simulink model "splittedMCU"  (R2021b)
settings: Solver=ode23tb  StartTime=0.0  StopTime=0.06  MaxStep=2.5e-7  RelTol=1e-3  EnableMultiTasking=on
libraries: spsIGBTDiodeLib x6, spsVoltageMeasurementLib x4, spsCurrentMeasurementLib x3, spsMeanLib x3, spsSeriesRLCBranchLib x3, simulink x2, spsControlledVoltageSourceLib x1, spsTHDLib x1, spspowerguiLib x1
settings Model: Creator=Алексей  LastModifiedBy=Len_comp
settings SolverCC: ZeroCrossControl=DisableAll  ZeroCrossAlgorithm=Adaptive  AlgebraicLoopSolver=TrustRegion
settings DataIOCC: SaveFormat=Array  SaveOutput=off  DSMLogging=off  SaveTime=off  ReturnWorkspaceOutputs=off
settings OptimizationCC: LifeSpan=inf
settings DebuggingCC: UnderspecifiedInitializationDetection=Classic  MergeDetectMultiDrivingBlocksExec=none  SolverPrmCheckMsg=warning  AllowSymbolicDim=off  SFUnexpectedBacktrackingDiag=warning  SFNoUnconditionalDefaultTransitionDiag=warning  SFExecutionAtInitializationDiag=none  SFMachineParentedDataDiag=warning  ArithmeticOperatorsInVariantConditions=warning
settings HardwareCC: ProdBitPerPointer=32  ProdBitPerSizeT=32  ProdBitPerPtrDiffT=32  ProdLargestAtomicFloat=None  ProdIntDivRoundTo=Undefined  ProdEndianess=Unspecified  ProdWordSize=32  ProdHWDeviceType=32-bit Generic
settings ModelReferenceCC: PropagateSignalLabelsOutOfModel=off
settings SFSimCC: SimUseLocalCustomCode=off  CustomCodeUndefinedFunction=UseInterfaceOnly
settings RTWCC: RTWUseLocalCustomCode=off
settings CodeAppCC: StateflowObjectComments=on
settings GRTTargetCC: TargetLangStandard=C89/C90 (ANSI)
settings ConfigComp: CovMetricSettings=dw  CovSaveCumulativeToWorkspaceVar=on  CovSaveSingleToWorkspaceVar=on  CovExternalEMLEnable=off  CovSFcnEnable=off
settings SimscapeCC: SimscapeNormalizeSystem=off

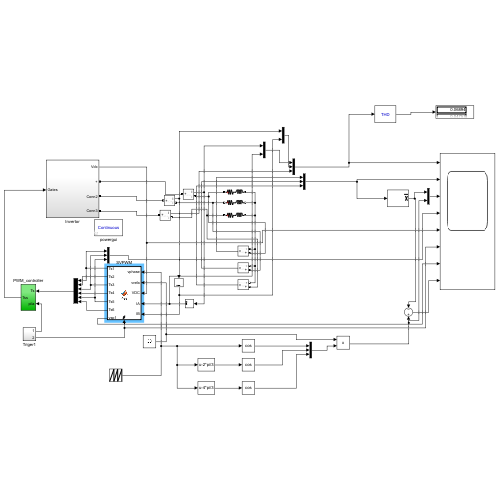
[thumbnail: Simulink's stored preview of the top-level diagram]
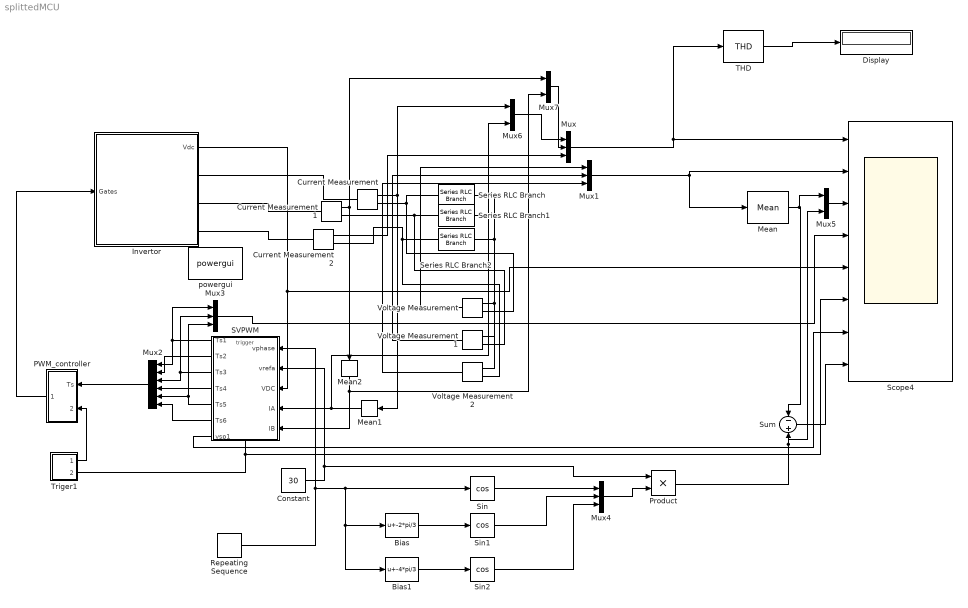
== system splittedMCU ==
  Bias : Bias  Bias=-2*pi/3
  Bias1 : Bias  Bias=-4*pi/3
  Constant : Constant  Value=30
  Current Measurement : spsCurrentMeasurementLib/Current Measurement  PhasorSimulation=off  OutputType=Complex  PSBequivalent=0
  Current Measurement1 : spsCurrentMeasurementLib/Current Measurement  PhasorSimulation=off  OutputType=Complex  PSBequivalent=0
  Current Measurement2 : spsCurrentMeasurementLib/Current Measurement  PhasorSimulation=off  OutputType=Complex  PSBequivalent=0
  Display : Display
  Invertor : Subsystem
  Mean : spsMeanLib/Mean  Freq=50e3  Vinit=0  Ts=0
  Mean1 : spsMeanLib/Mean  Freq=50e3  Vinit=0  Ts=0
  Mean2 : spsMeanLib/Mean  Freq=50e3  Vinit=0  Ts=0
  Mux{,1,3..4} (4 alike) : Mux  Inputs=3
  Mux2 : Mux  Inputs=6
  Mux5 : Mux  Inputs=2
  Mux6 : Mux  Inputs=2
  Mux7 : Mux  Inputs=2
  PWM_controller : Subsystem
  Product : Product
  Repeating Sequence : simulink/Sources/Repeating Sequence  rep_seq_t=[0 0.02]  rep_seq_y=[0 2*pi]
  SVPWM : MATLAB Function  TreatAsAtomicUnit=on
  Scope4 : Scope  NumInputPorts=8
  Series RLC Branch : spsSeriesRLCBranchLib/Series RLC Branch  LConnTagsString=__new0  RConnTagsString=__new0  BranchType=RL  Resistance=1  Inductance=35e-6  SetiL0=off  InitialCurrent=236  Capacitance=1e-6  Setx0=off  InitialVoltage=0  Measurements=None
  Series RLC Branch1 : spsSeriesRLCBranchLib/Series RLC Branch  LConnTagsString=__new0  RConnTagsString=__new0  BranchType=RL  Resistance=1  Inductance=35e-6  SetiL0=off  InitialCurrent=236  Capacitance=1e-6  Setx0=off  InitialVoltage=0  Measurements=None
  Series RLC Branch2 : spsSeriesRLCBranchLib/Series RLC Branch  LConnTagsString=__new0  RConnTagsString=__new0  BranchType=RL  Resistance=1  Inductance=35e-6  SetiL0=off  InitialCurrent=-236  Capacitance=1e-6  Setx0=off  InitialVoltage=0  Measurements=None
  Sin : Trigonometry  Operator=cos
  Sin1 : Trigonometry  Operator=cos
  Sin2 : Trigonometry  Operator=cos
  Sum : Sum  Inputs=-+
  THD : spsTHDLib/THD  Freq=50  Ts=0
      settings: SourceProductBaseCode=PS
  Triger1 : Subsystem
  Voltage Measurement : spsVoltageMeasurementLib/Voltage Measurement  PhasorSimulation=off  OutputType=Complex  PSBequivalent=0
  Voltage Measurement1 : spsVoltageMeasurementLib/Voltage Measurement  PhasorSimulation=off  OutputType=Complex  PSBequivalent=0
  Voltage Measurement2 : spsVoltageMeasurementLib/Voltage Measurement  PhasorSimulation=off  OutputType=Complex  PSBequivalent=0
  powergui : spspowerguiLib/powergui  Priority=1  SimulationMode=Continuous  SampleTime=50e-6  frequency=60  Iterations=50  frequencyindice=0  Pbase=100e6  ErrMax=1e-4  UnitsV=kV  UnitsW=MW  buscounter=0  FunctionMessages=off  echomessages=off  EnableUseOfTLC=off  CurrentSourceSwitches=on  DisableSnubberDevices=off  DisableRonSwitches=off  DisableVfSwitches=off  DisplayEquations=off  AutomaticDiscreteSolvers=off  SolverType=Tustin  Interpol=off  ExternalGateDelay=off  methode=off  Ts=0  x0status=blocks  SPID=off  SwTol=0  HookPort=off  NonlinearTolerance=1e-4  nMaxIteration=100  ContinueOnMaxIteration=off  RestoreLinks=warning  ResistiveCurrentMeasurement=off  Frange=[0:2:500]  Ylog=off  Xlog=on  ShowGrid=off  save=off  variable=ZData  structure=SD2  ZoomFFT=on  StartTime=0.7  cycles=10  DisplayStyle=4  fundamental=382  FreqAxis=off  MaxFrequency=50000  frequencyindicesteady=1  RmsSteady=1  display=off
  wires:
  Mux2/1 -> PWM_controller/1(Ts)
  Triger1/1(1) -> PWM_controller/2(pila)
  PWM_controller/1(Tss) -> Invertor/1(Gates)
  Invertor/1(Vdc) -> Scope4/5, SVPWM/3(VDC)
  SVPWM/1(Ts1) -> Mux2/1, Mux3/1
  SVPWM/2(Ts2) -> Mux2/2
  SVPWM/3(Ts3) -> Mux2/3, Mux3/2
  SVPWM/4(Ts4) -> Mux2/4
  SVPWM/5(Ts5) -> Mux3/3, Mux2/5
  SVPWM/6(Ts6) -> Mux2/6
  Triger1/2(2) -> Scope4/6, SVPWM/Trigger
  Current Measurement/1 -> Mux6/1, Mean1/1
  Current Measurement1/1 -> Mux7/1, Mean2/1
  Constant/1 -> Product/1, SVPWM/2(vrefa)
  Repeating Sequence/1 -> Bias1/1, Bias/1, Sin/1, SVPWM/1(vphase)
  Current Measurement2/1 -> Mux/3
  Mux/1 -> THD/1, Scope4/1
  Voltage Measurement/1 -> Mux1/1
  Voltage Measurement1/1 -> Mux1/2
  Voltage Measurement2/1 -> Mux1/3
  Mean/1 -> Mux5/1, Sum/1
  Mux1/1 -> Mean/1, Scope4/2
  Mux3/1 -> Scope4/4
  SVPWM/7(vsp1) -> Scope4/7
  THD/1 -> Display/1
  Bias/1 -> Sin1/1
  Bias1/1 -> Sin2/1
  Sin/1 -> Mux4/1
  Sin1/1 -> Mux4/2
  Sin2/1 -> Mux4/3
  Mux4/1 -> Product/2
  Product/1 -> Mux5/2, Sum/2
  Sum/1 -> Scope4/8
  Mean1/1 -> Mux6/2, SVPWM/4(IA)
  Mean2/1 -> SVPWM/5(IB), Mux7/2
  Mux5/1 -> Scope4/3
  Mux6/1 -> Mux/1
  Mux7/1 -> Mux/2
  connections:
  Current Measurement/LConn1 -- Invertor/RConn1
  Invertor/RConn3 -- Current Measurement2/LConn1
  Invertor/RConn2 -- Current Measurement1/LConn1
  Voltage Measurement/LConn2 -- Voltage Measurement2/LConn2 -- Voltage Measurement1/LConn2 -- Series RLC Branch/RConn1 -- Series RLC Branch1/RConn1 -- Series RLC Branch2/RConn1
  Current Measurement/RConn1 -- Series RLC Branch/LConn1 -- Voltage Measurement/LConn1
  Current Measurement1/RConn1 -- Series RLC Branch1/LConn1 -- Voltage Measurement1/LConn1
  Current Measurement2/RConn1 -- Series RLC Branch2/LConn1 -- Voltage Measurement2/LConn1

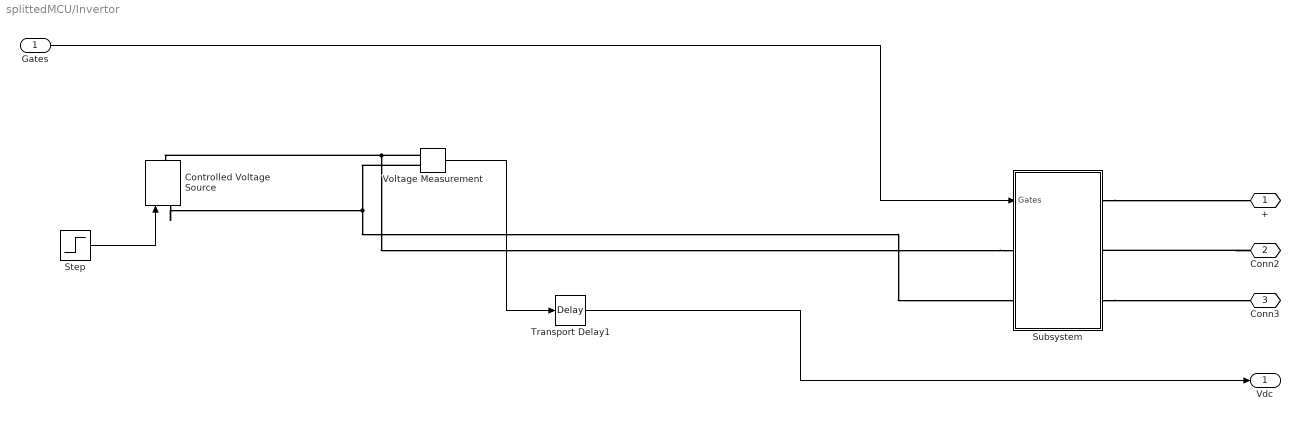
== system splittedMCU/Invertor ==
  Gates : Inport
  Controlled Voltage Source : spsControlledVoltageSourceLib/Controlled Voltage Source  Initialize=on  Source_Type=AC  Amplitude=0  Phase=0  Frequency=0  Measurements=None
  Step : Step  Time=6  Before=100  After=300  SampleTime=0
  Subsystem : Subsystem
  Transport Delay1 : TransportDelay  DelayTime=26e-6
  Voltage Measurement : spsVoltageMeasurementLib/Voltage Measurement  PhasorSimulation=off  OutputType=Complex  PSBequivalent=0
  + : PMIOPort  Side=Right
  Conn2 : PMIOPort  Port=2  Side=Right
  Conn3 : PMIOPort  Port=3  Side=Right
  Vdc : Outport  VectorParamsAs1DForOutWhenUnconnected=off
  wires:
  Voltage Measurement/1 -> Transport Delay1/1
  Transport Delay1/1 -> Vdc/1
  Step/1 -> Controlled Voltage Source/1
  Gates/1 -> Subsystem/1(Gates)
  connections:
  Subsystem/LConn1 -- Controlled Voltage Source/RConn1 -- Voltage Measurement/LConn1
  Subsystem/RConn1 -- +/RConn1
  Conn2/RConn1 -- Subsystem/RConn2
  Subsystem/RConn3 -- Conn3/RConn1
  Voltage Measurement/LConn2 -- Controlled Voltage Source/LConn1 -- Subsystem/LConn2

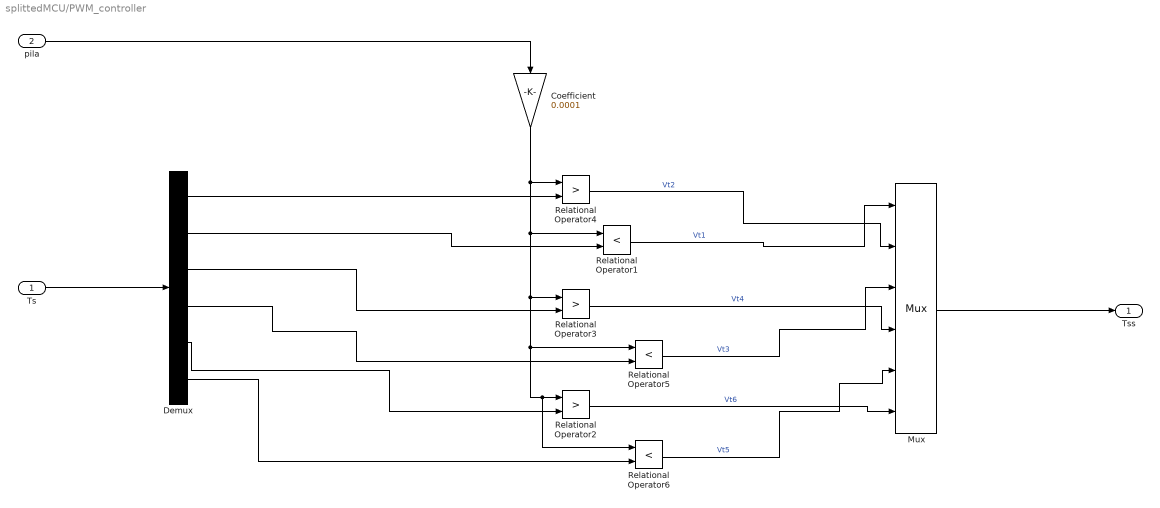
== system splittedMCU/PWM_controller ==
  Ts : Inport
  pila : Inport  Port=2
  Coefficient : Gain  Gain=0.0001
  Demux : Demux  Outputs=6
  Mux : Mux  Inputs=6
  Relational Operator1 : RelationalOperator  Operator=<  OutDataTypeStr=boolean  RndMeth=Nearest
  Relational Operator2 : RelationalOperator  Operator=>  OutDataTypeStr=boolean  RndMeth=Nearest
  Relational Operator3 : RelationalOperator  Operator=>  OutDataTypeStr=boolean  RndMeth=Nearest
  Relational Operator4 : RelationalOperator  Operator=>  OutDataTypeStr=boolean  RndMeth=Nearest
  Relational Operator5 : RelationalOperator  Operator=<  OutDataTypeStr=boolean  RndMeth=Nearest
  Relational Operator6 : RelationalOperator  Operator=<  OutDataTypeStr=boolean  RndMeth=Nearest
  Tss : Outport  VectorParamsAs1DForOutWhenUnconnected=off
  wires:
  Relational Operator4/1 -> Mux/2  "Vt2"
  Demux/3 -> Relational Operator3/2
  Demux/5 -> Relational Operator2/2
  Relational Operator3/1 -> Mux/4  "Vt4"
  Relational Operator2/1 -> Mux/6  "Vt6"
  Ts/1 -> Demux/1
  Coefficient/1 -> Relational Operator1/1, Relational Operator3/1, Relational Operator5/1, Relational Operator6/1, Relational Operator2/1, Relational Operator4/1
  Relational Operator1/1 -> Mux/1  "Vt1"
  Relational Operator5/1 -> Mux/3  "Vt3"
  Relational Operator6/1 -> Mux/5  "Vt5"
  Demux/2 -> Relational Operator1/2
  Demux/4 -> Relational Operator5/2
  Demux/6 -> Relational Operator6/2
  Demux/1 -> Relational Operator4/2
  pila/1 -> Coefficient/1
  Mux/1 -> Tss/1

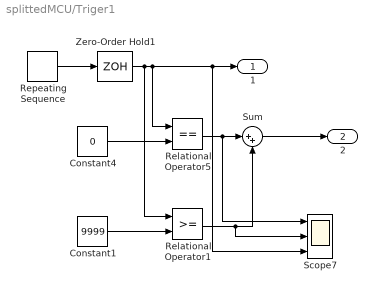
== system splittedMCU/Triger1 ==
  Constant1 : Constant  Value=9999
  Constant4 : Constant  Value=0
  Relational Operator1 : RelationalOperator  OutDataTypeStr=boolean  RndMeth=Nearest
  Relational Operator5 : RelationalOperator  Operator===  OutDataTypeStr=boolean  RndMeth=Nearest
  Repeating Sequence : simulink/Sources/Repeating Sequence  rep_seq_t=[0 10e-6 20e-6]  rep_seq_y=[0 10000 0]
  Scope7 : Scope  NumInputPorts=3
  Sum : Sum  Inputs=|++
  Zero-Order Hold1 : ZeroOrderHold  SampleTime=2.5e-8
  1 : Outport  VectorParamsAs1DForOutWhenUnconnected=off
  2 : Outport  Port=2  VectorParamsAs1DForOutWhenUnconnected=off
  wires:
  Zero-Order Hold1/1 -> Relational Operator1/1, Relational Operator5/1, Scope7/3, 1/1
  Repeating Sequence/1 -> Zero-Order Hold1/1
  Constant4/1 -> Relational Operator5/2
  Sum/1 -> 2/1
  Constant1/1 -> Relational Operator1/2
  Relational Operator5/1 -> Scope7/1, Sum/1
  Relational Operator1/1 -> Scope7/2, Sum/2

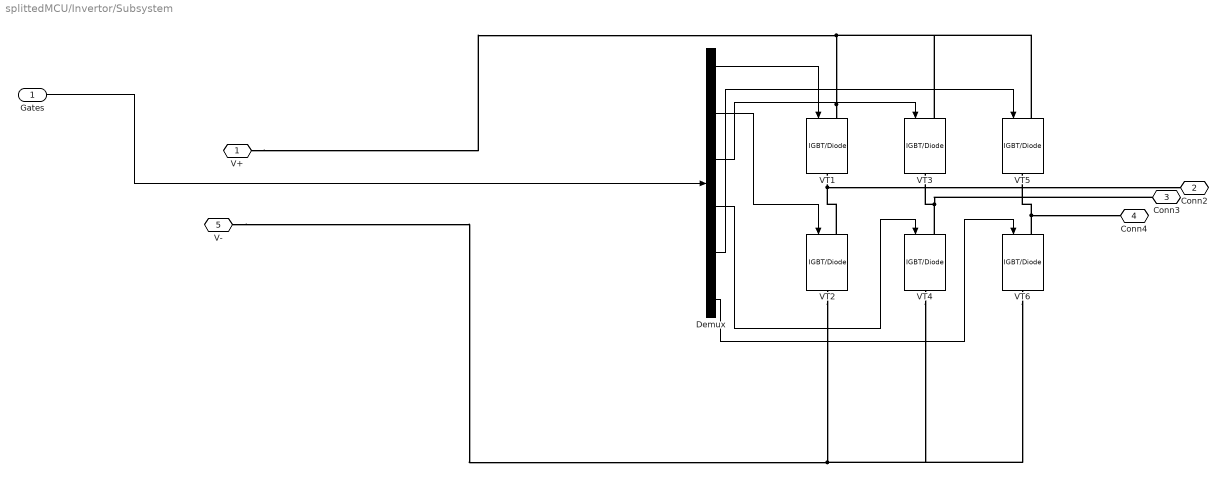
== system splittedMCU/Invertor/Subsystem ==
  Gates : Inport
  Demux : Demux  Outputs=6
  VT{1..6} (6 alike) : spsIGBTDiodeLib/IGBT//Diode  Ron=1e-3  Rs=1e5  Cs=inf  Measurements=off
  V+ : PMIOPort  Side=Left
  Conn2 : PMIOPort  Port=2  Side=Right
  Conn3 : PMIOPort  Port=3  Side=Right
  Conn4 : PMIOPort  Port=4  Side=Right
  V- : PMIOPort  Port=5  Side=Left
  wires:
  Demux/4 -> VT4/1
  Demux/2 -> VT2/1
  Demux/5 -> VT5/1
  Demux/3 -> VT3/1
  Demux/6 -> VT6/1
  Demux/1 -> VT1/1
  Gates/1 -> Demux/1
  connections:
  VT6/LConn1 -- Conn4/RConn1 -- VT5/RConn1
  V-/RConn1 -- VT2/RConn1 -- VT4/RConn1 -- VT6/RConn1
  VT4/LConn1 -- Conn3/RConn1 -- VT3/RConn1
  VT1/LConn1 -- V+/RConn1 -- VT5/LConn1 -- VT3/LConn1
  VT2/LConn1 -- Conn2/RConn1 -- VT1/RConn1

== matlab function splittedMCU/SVPWM ==
  data: vphase input; vrefa input; VDC input; IA input; IB input; Ts1 output; Ts2 output; Ts3 output; Ts4 output; Ts5 output; Ts6 output; vsp1 output
  events: trigger input RISING_EDGE_EVENT
function [Ts1,Ts2,Ts3,Ts4,Ts5,Ts6,vsp1] = fcn(vphase,vrefa,VDC,IA,IB)
%время 1/2 ШИМ периода
dt=10e-6;


%алгоритм формирования векторной ШИМ  мертвым веменем dead [мкс]
dead=1.5;

compensate = 1;


vsp1 = vphase;

dead=dead/(dt*1e6);
a=vphase;
v2=vrefa*1.5;
if a>=0 && a<pi/3 
    n=1;
elseif  a>=pi/3 && a<2*pi/3 
    n=2;
elseif  a>=2*pi/3 && a<pi 
    n=3;
elseif  a>=pi && a<4*pi/3 
    n=4;
elseif  a>=4*pi/3 && a<5*pi/3 
    n=5;
else n=6;

end

a_cor=a-(n-1)*pi/3;

T1 = (v2/VDC)*sin(pi/3-a_cor)/sin(pi/3);
T2 = (v2/VDC)*sin(a_cor)/sin(pi/3);
T0=1-T1-T2;
Ta1=0; Ta3=0; Ta5=0; 
switch n
    case 1
        
        Ta1=T1+T2+T0/2;
        
        Ta3=T2+T0/2;
       
        Ta5=T0/2;
       
    case 2
        
        Ta1=T1+T0/2;
        
        Ta3=T1+T2+T0/2;
    
        Ta5=T0/2;       
        
    case 3
        
        Ta1=T0/2;
       
        Ta3=T1+T2+T0/2;
       
        Ta5=T2+T0/2;    
        
    case 4
        
        Ta1=T0/2;
       
        Ta3=T1+T0/2;
       
        Ta5=T1+T2+T0/2;   
       
    case 5
        
        Ta1=T2+T0/2;
        
        Ta3=T0/2;
        
        Ta5=T1+T2+T0/2;     
        
    case 6
        
        Ta1=T1+T2+T0/2;
        
        Ta3=T0/2;
     
        Ta5=T1+T0/2;    
        
end;


Ts1=(Ta1) + dead/2; 
Ts3=(Ta3) + dead/2; 
Ts5=(Ta5) + dead/2;
Ts2=(Ta1) - dead/2; 
Ts4=(Ta3) - dead/2; 
Ts6=(Ta5) - dead/2;

k = 0.5;
ilim = 3;

if compensate == 1
    if (IA > ilim) 
        Ts1=Ts1+dead*k;
        Ts2=Ts2+dead*k;
    elseif(IA < -ilim)
        Ts1=Ts1-dead*k;
        Ts2=Ts2-dead*k;           
    end
    if (IB > ilim) 
        Ts3=Ts3+dead*k;
        Ts4=Ts4+dead*k; 
    elseif(IB < -ilim)
        Ts3=Ts3-dead*k;
        Ts4=Ts4-dead*k; 
    end  
    if ((-IA-IB) > ilim) 
        Ts5=Ts5+dead*k;
        Ts6=Ts6+dead*k;
    elseif((-IA - IB) < -ilim)
        Ts5=Ts5-dead*k;
        Ts6=Ts6-dead*k;           
    end
end

return;
